simulink model "as_labor03_u_motor_dc"  (R2020b)
settings: Solver=ode15s  StartTime=0.0  StopTime=0.6  RelTol=1e-3
undefined symbols (not defined in the file): cr, J, ke, km, L, R, Rs
settings Model: Creator=jan  LastModifiedBy=jan
settings HardwareCC: ProdBitPerLong=64  ProdHWDeviceType=Intel->x86-64 (Linux 64)

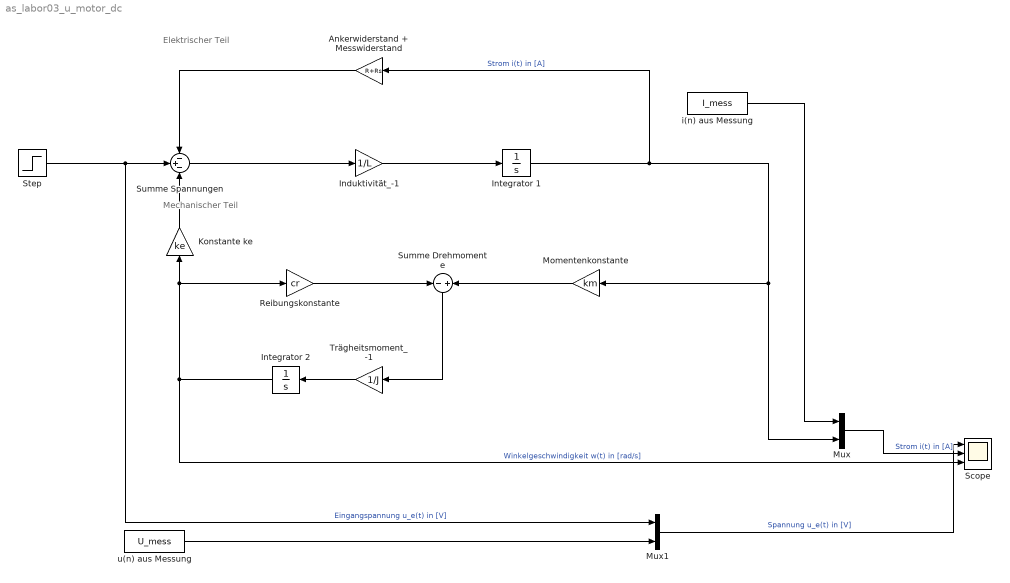
== system as_labor03_u_motor_dc ==
  note: Elektrischer Teil
  note: Mechanischer Teil
  Ankerwiderstand + Messwiderstand : Gain  Gain=R+Rs
  Induktivität_-1 : Gain  Gain=1/L
  Integrator 1 : Integrator
  Integrator 2 : Integrator
  Konstante ke : Gain  Gain=ke
  Momentenkonstante : Gain  Gain=km
  Mux : Mux  Inputs=2
  Mux1 : Mux  Inputs=2
  Reibungskonstante : Gain  Gain=cr
  Scope : Scope  NumInputPorts=3
  Step : Step  Time=0.048  After=8.2  SampleTime=0.001
  Summe Drehmomente : Sum  Inputs=-|+
  Summe Spannungen : Sum  Inputs=-+-
  Trägheitsmoment_-1 : Gain  Gain=1/J
  i(n) aus Messung : FromWorkspace  VariableName=I_mess  Interpolate=off  ZeroCross=off  OutputAfterFinalValue=Holding final value
  u(n) aus Messung : FromWorkspace  VariableName=U_mess  Interpolate=off  ZeroCross=off  OutputAfterFinalValue=Holding final value
  wires:
  Summe Spannungen/1 -> Induktivität_-1/1
  Induktivität_-1/1 -> Integrator 1/1
  Integrator 1/1 -> Mux/2, Momentenkonstante/1, Ankerwiderstand + Messwiderstand/1  "Strom i(t) in [A]"
  Reibungskonstante/1 -> Summe Drehmomente/1
  Momentenkonstante/1 -> Summe Drehmomente/2
  Ankerwiderstand + Messwiderstand/1 -> Summe Spannungen/1
  Konstante ke/1 -> Summe Spannungen/3
  Summe Drehmomente/1 -> Trägheitsmoment_-1/1
  Trägheitsmoment_-1/1 -> Integrator 2/1
  Integrator 2/1 -> Scope/3, Reibungskonstante/1, Konstante ke/1  "Winkelgeschwindigkeit w(t) in [rad/s]"
  Step/1 -> Mux1/1, Summe Spannungen/2  "Eingangspannung u_e(t) in [V]"
  i(n) aus Messung/1 -> Mux/1
  u(n) aus Messung/1 -> Mux1/2
  Mux1/1 -> Scope/1  "Spannung u_e(t) in [V]"
  Mux/1 -> Scope/2  "Strom i(t) in [A]"
